simulink model "Vertical_Fin_Model_SAAM"  (R2018a)
settings: Solver=FixedStepAuto  StartTime=0.0  StopTime=10.0  FixedStep=dt  RelTol=1e-3
values from neighbouring files (symbols this model uses):
  A_vt = 2.5    [airplane_ic_constants.m]
  CD0_vt = 0.01    [airplane_ic_constants.m]
  CDfp_vt = 1    [airplane_ic_constants.m]
  CL0_vt = 0    [airplane_ic_constants.m]
  CLmax_vt = 1.1    [airplane_ic_constants.m]
  K_vt = 0.084    [airplane_ic_constants.m]
  n_vt = 1.6    [airplane_ic_constants.m]
  S_vt = 1.3    [airplane_ic_constants.m]
  tauRud = 0.7    [airplane_ic_constants.m]
libraries: simulink x3
settings Model: Creator=Kyle  LastModifiedBy=Kyle

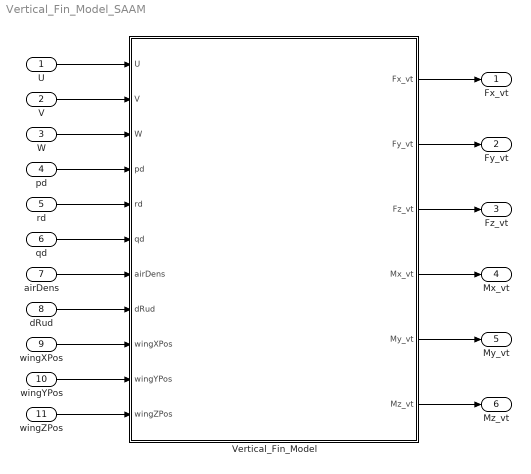
== system Vertical_Fin_Model_SAAM ==
  U : Inport
  V : Inport  Port=2
  W : Inport  Port=3
  pd : Inport  Port=4
  rd : Inport  Port=5
  qd : Inport  Port=6
  airDens : Inport  Port=7
  dRud : Inport  Port=8
  wingXPos : Inport  Port=9
  wingYPos : Inport  Port=10
  wingZPos : Inport  Port=11
  Vertical_Fin_Model : Subsystem
  Fx_vt : Outport
  Fy_vt : Outport  Port=2
  Fz_vt : Outport  Port=3
  Mx_vt : Outport  Port=4
  My_vt : Outport  Port=5
  Mz_vt : Outport  Port=6
  wires:
  U/1 -> Vertical_Fin_Model/1(U)
  V/1 -> Vertical_Fin_Model/2(V)
  W/1 -> Vertical_Fin_Model/3(W)
  pd/1 -> Vertical_Fin_Model/4(pd)
  wingXPos/1 -> Vertical_Fin_Model/9(wingXPos)
  wingYPos/1 -> Vertical_Fin_Model/10(wingYPos)
  wingZPos/1 -> Vertical_Fin_Model/11(wingZPos)
  dRud/1 -> Vertical_Fin_Model/8(dRud)
  rd/1 -> Vertical_Fin_Model/5(rd)
  qd/1 -> Vertical_Fin_Model/6(qd)
  airDens/1 -> Vertical_Fin_Model/7(airDens)
  Vertical_Fin_Model/4(Mx_vt) -> Mx_vt/1
  Vertical_Fin_Model/6(Mz_vt) -> Mz_vt/1
  Vertical_Fin_Model/5(My_vt) -> My_vt/1
  Vertical_Fin_Model/2(Fy_vt) -> Fy_vt/1
  Vertical_Fin_Model/1(Fx_vt) -> Fx_vt/1
  Vertical_Fin_Model/3(Fz_vt) -> Fz_vt/1

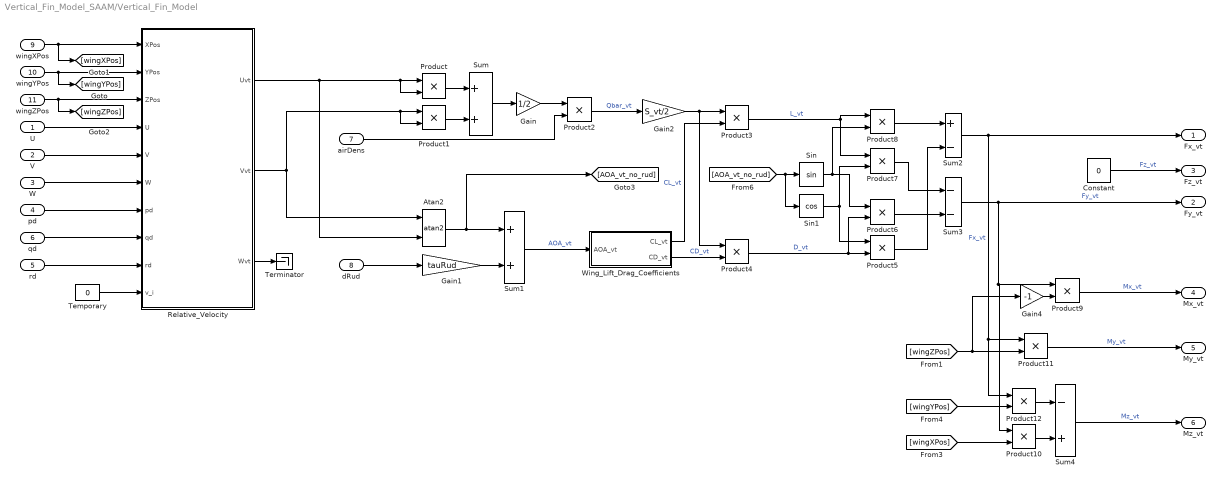
== system Vertical_Fin_Model_SAAM/Vertical_Fin_Model ==
  U : Inport
  V : Inport  Port=2
  W : Inport  Port=3
  pd : Inport  Port=4
  rd : Inport  Port=5
  qd : Inport  Port=6
  airDens : Inport  Port=7
  dRud : Inport  Port=8
  wingXPos : Inport  Port=9
  wingYPos : Inport  Port=10
  wingZPos : Inport  Port=11
  Atan2 : Trigonometry  Operator=atan2
  Constant : Constant  Value=0
  Gain : Gain  Gain=1/2
  Gain1 : Gain  Gain=tauRud
  Gain2 : Gain  Gain=S_vt/2
  Gain4 : Gain  Gain=-1
  Product{,1..12} (13 alike) : Product
  Relative_Velocity : Subsystem
  Sin : Trigonometry
  Sin1 : Trigonometry  Operator=cos
  Sum : Sum
  Sum1 : Sum
  Sum2 : Sum  Inputs=+-
  Sum3 : Sum  Inputs=--
  Sum4 : Sum  Inputs=-+
  Temporary : Constant  Value=0
  Terminator : Terminator
  Wing_Lift_Drag_Coefficients : Subsystem
  Fx_vt : Outport
  Fy_vt : Outport  Port=2
  Fz_vt : Outport  Port=3
  Mx_vt : Outport  Port=4
  My_vt : Outport  Port=5
  Mz_vt : Outport  Port=6
  wires:
  wingYPos/1 -> [wingYPos], Relative_Velocity/2(YPos)
  wingZPos/1 -> [wingZPos], Relative_Velocity/3(ZPos)
  U/1 -> Relative_Velocity/4(U)
  V/1 -> Relative_Velocity/5(V)
  W/1 -> Relative_Velocity/6(W)
  pd/1 -> Relative_Velocity/7(pd)
  rd/1 -> Relative_Velocity/9(rd)
  qd/1 -> Relative_Velocity/8(qd)
  Sum/1 -> Gain/1
  Product/1 -> Sum/1
  Product1/1 -> Sum/2
  Gain/1 -> Product2/1
  airDens/1 -> Product2/2
  Relative_Velocity/1(Uvt) -> Atan2/2, Product/2, Product/1
  dRud/1 -> Gain1/1
  Gain1/1 -> Sum1/2
  Atan2/1 -> [AOA_vt_no_rud], Sum1/1
  Product2/1 -> Gain2/1  "Qbar_vt"
  Sum1/1 -> Wing_Lift_Drag_Coefficients/1(AOA_vt)  "AOA_vt"
  Gain2/1 -> Product4/1, Product3/1
  Wing_Lift_Drag_Coefficients/1(CL_vt) -> Product3/2  "CL_vt"
  Wing_Lift_Drag_Coefficients/2("CD_vt ") -> Product4/2  "CD_vt"
  Product4/1 -> Product5/2, Product6/2  "D_vt"
  [AOA_vt_no_rud] -> Sin1/1, Sin/1
  Sin1/1 -> Product5/1, Product7/2
  Sin/1 -> Product8/2, Product6/1
  Product3/1 -> Product8/1, Product7/1  "L_vt"
  Product8/1 -> Sum2/1
  Product5/1 -> Sum2/2
  Product7/1 -> Sum3/1
  Product6/1 -> Sum3/2
  Sum3/1 -> Fy_vt/1, Product10/1, Product9/1  "Fy_vt"
  wingXPos/1 -> [wingXPos], Relative_Velocity/1(XPos)
  Product9/1 -> Mx_vt/1  "Mx_vt"
  Sum2/1 -> Fx_vt/1, Product11/1, Product12/1  "Fx_vt"
  [wingZPos] -> Gain4/1, Product11/2
  Product11/1 -> My_vt/1  "My_vt"
  Product12/1 -> Sum4/1
  Sum4/1 -> Mz_vt/1  "Mz_vt"
  Temporary/1 -> Relative_Velocity/10(v_i)
  Relative_Velocity/3(Wvt) -> Terminator/1
  Relative_Velocity/2(Vvt) -> Atan2/1, Product1/2, Product1/1
  Constant/1 -> Fz_vt/1  "Fz_vt"
  Gain4/1 -> Product9/2
  [wingYPos] -> Product12/2
  Product10/1 -> Sum4/2
  [wingXPos] -> Product10/2

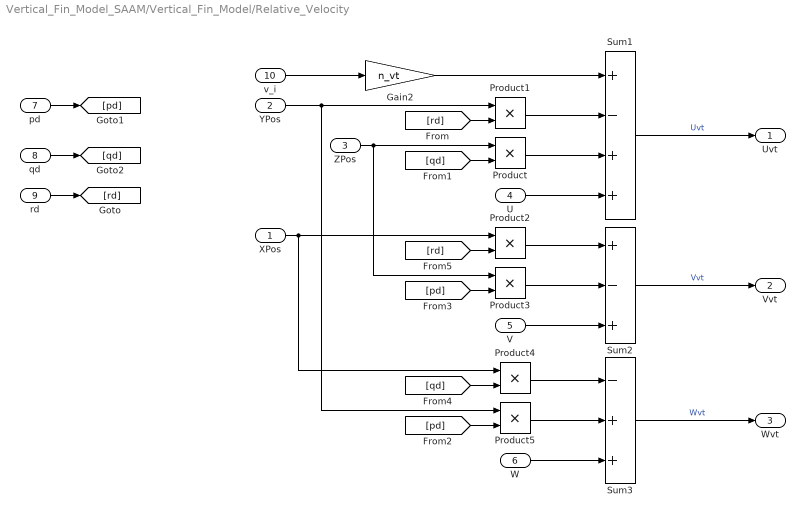
== system Vertical_Fin_Model_SAAM/Vertical_Fin_Model/Relative_Velocity ==
  XPos : Inport
  YPos : Inport  Port=2
  ZPos : Inport  Port=3
  U : Inport  Port=4
  V : Inport  Port=5
  W : Inport  Port=6
  pd : Inport  Port=7
  qd : Inport  Port=8
  rd : Inport  Port=9
  v_i : Inport  Port=10
  Gain2 : Gain  Gain=n_vt
  Product{,1..5} (6 alike) : Product
  Sum1 : Sum  Inputs=+-++
  Sum2 : Sum  Inputs=+-+
  Sum3 : Sum  Inputs=-++
  Uvt : Outport
  Vvt : Outport  Port=2
  Wvt : Outport  Port=3
  wires:
  ZPos/1 -> Product3/1, Product/1
  Product/1 -> Sum1/3
  U/1 -> Sum1/4
  [rd] -> Product1/2
  Product1/1 -> Sum1/2
  rd/1 -> [rd]
  pd/1 -> [pd]
  qd/1 -> [qd]
  [qd] -> Product/2
  V/1 -> Sum2/3
  Sum2/1 -> Vvt/1  "Vvt"
  Sum3/1 -> Wvt/1  "Wvt"
  W/1 -> Sum3/3
  Product3/1 -> Sum2/2
  Product2/1 -> Sum2/1
  XPos/1 -> Product4/1, Product2/1
  YPos/1 -> Product5/1, Product1/1
  Product5/1 -> Sum3/2
  Product4/1 -> Sum3/1
  [pd] -> Product5/2
  [pd] -> Product3/2
  [rd] -> Product2/2
  [qd] -> Product4/2
  Sum1/1 -> Uvt/1  "Uvt"
  v_i/1 -> Gain2/1
  Gain2/1 -> Sum1/1

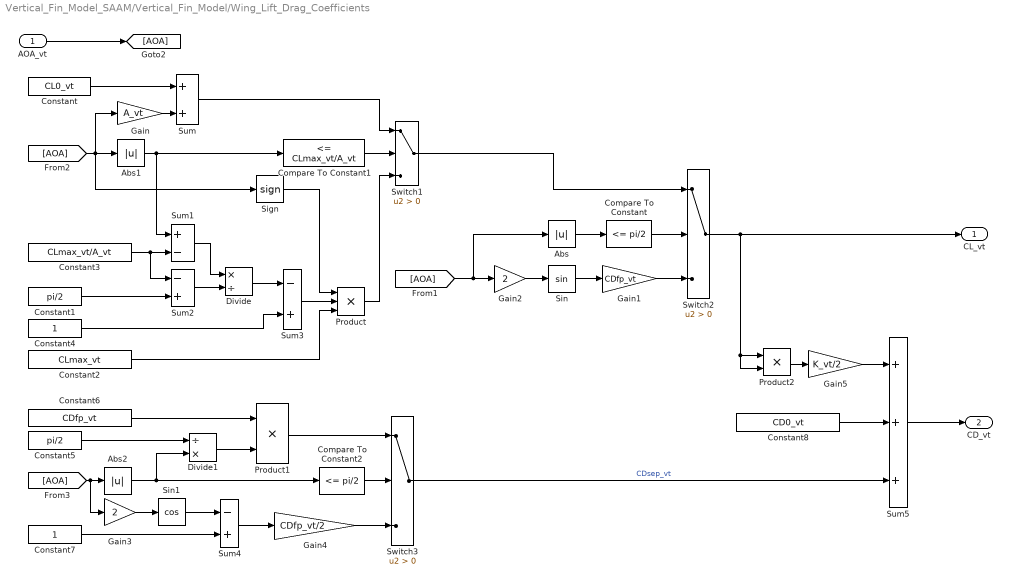
== system Vertical_Fin_Model_SAAM/Vertical_Fin_Model/Wing_Lift_Drag_Coefficients ==
  AOA_vt : Inport
  Abs : Abs
  Abs1 : Abs
  Abs2 : Abs
  Compare To Constant : simulink/Logic and Bit Operations/Compare To Constant  relop=<=  const=pi/2  OutDataTypeStr=boolean
  Compare To Constant1 : simulink/Logic and Bit Operations/Compare To Constant  relop=<=  const=CLmax_vt/A_vt  OutDataTypeStr=boolean
  Compare To Constant2 : simulink/Logic and Bit Operations/Compare To Constant  relop=<=  const=pi/2  OutDataTypeStr=boolean
  Constant : Constant  Value=CL0_vt
  Constant1 : Constant  Value=pi/2
  Constant2 : Constant  Value=CLmax_vt
  Constant3 : Constant  Value=CLmax_vt/A_vt
  Constant4 : Constant
  Constant5 : Constant  Value=pi/2
  Constant6 : Constant  Value=CDfp_vt
  Constant7 : Constant
  Constant8 : Constant  Value=CD0_vt
  Divide : Product  Inputs=*/
  Divide1 : Product  Inputs=/*
  Gain : Gain  Gain=A_vt
  Gain1 : Gain  Gain=CDfp_vt
  Gain2 : Gain  Gain=2
  Gain3 : Gain  Gain=2
  Gain4 : Gain  Gain=CDfp_vt/2
  Gain5 : Gain  Gain=K_vt/2
  Product : Product  Inputs=3
  Product1 : Product
  Product2 : Product
  Sign : Signum
  Sin : Trigonometry
  Sin1 : Trigonometry  Operator=cos
  Sum : Sum
  Sum1 : Sum  Inputs=+-
  Sum2 : Sum  Inputs=-+
  Sum3 : Sum  Inputs=-+
  Sum4 : Sum  Inputs=-+
  Sum5 : Sum  Inputs=+++
  Switch1 : Switch  Criteria=u2 > Threshold
  Switch2 : Switch  Criteria=u2 > Threshold
  Switch3 : Switch  Criteria=u2 > Threshold
  CL_vt : Outport
  "CD_vt " : Outport  Port=2
  wires:
  Compare To Constant/1 -> Switch2/2
  AOA_vt/1 -> [AOA]
  [AOA] -> Gain2/1, Abs/1
  Abs/1 -> Compare To Constant/1
  Abs1/1 -> Sum1/1, Compare To Constant1/1
  [AOA] -> Sign/1, Abs1/1, Gain/1
  Compare To Constant1/1 -> Switch1/2
  Constant/1 -> Sum/1
  Gain/1 -> Sum/2
  Sum/1 -> Switch1/1
  Constant3/1 -> Sum2/1, Sum1/2
  Constant1/1 -> Sum2/2
  Sum1/1 -> Divide/1
  Sum2/1 -> Divide/2
  Constant4/1 -> Sum3/2
  Divide/1 -> Sum3/1
  Sum3/1 -> Product/2
  Constant2/1 -> Product/3
  Product/1 -> Switch1/3
  Switch1/1 -> Switch2/1
  Gain1/1 -> Switch2/3
  Switch2/1 -> CL_vt/1, Product2/1, Product2/2
  Sin/1 -> Gain1/1
  Gain2/1 -> Sin/1
  [AOA] -> Gain3/1, Abs2/1
  Compare To Constant2/1 -> Switch3/2
  Abs2/1 -> Compare To Constant2/1, Divide1/2
  Constant5/1 -> Divide1/1
  Divide1/1 -> Product1/2
  Product1/1 -> Switch3/1
  Constant6/1 -> Product1/1
  Sin1/1 -> Sum4/1
  Gain3/1 -> Sin1/1
  Constant7/1 -> Sum4/2
  Sum4/1 -> Gain4/1
  Gain4/1 -> Switch3/3
  Switch3/1 -> Sum5/3  "CDsep_vt"
  Product2/1 -> Gain5/1
  Gain5/1 -> Sum5/1
  Sum5/1 -> "CD_vt "/1
  Constant8/1 -> Sum5/2
  Sign/1 -> Product/1
